simulink subsystem "PID_MotorFB"  (R2024a)
settings: Solver=VariableStepAuto  StartTime=0.0  StopTime=10.0  RelTol=1e-3
undefined symbols (not defined in the file or in its folder): Ki_m, Kp_m, motorFBRate, Tw_m
settings Model: Creator=Peter  LastModifiedBy=Peter

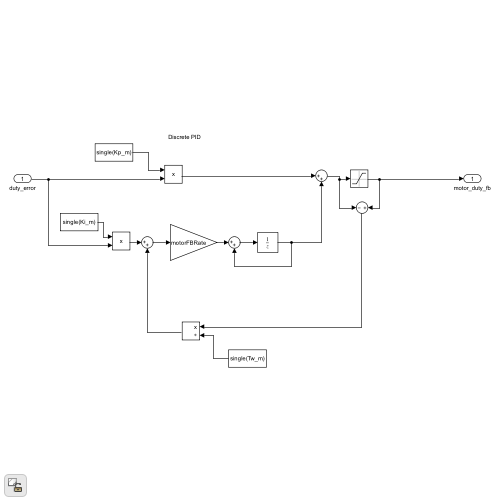
[thumbnail: Simulink's stored preview of the top-level diagram]
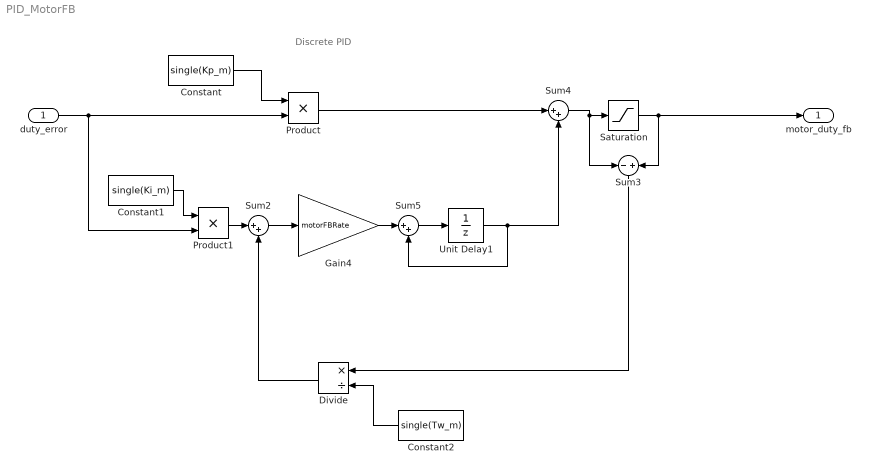
== system PID_MotorFB ==
  note: Discrete PID
  duty_error : Inport
  Constant : Constant  Value=single(Kp_m)
  Constant1 : Constant  Value=single(Ki_m)
  Constant2 : Constant  Value=single(Tw_m)
  Divide : Product  Inputs=*/
  Gain4 : Gain  Gain=motorFBRate
  Product : Product
  Product1 : Product
  Saturation : Saturate  UpperLimit=1  LowerLimit=0
  Sum2 : Sum  Inputs=|++
  Sum3 : Sum  Inputs=-|+
  Sum4 : Sum  Inputs=|++
  Sum5 : Sum  Inputs=|++
  Unit Delay1 : UnitDelay  SampleTime=motorFBRate  HasFrameUpgradeWarning=on
  motor_duty_fb : Outport
  wires:
  Sum5/1 -> Unit Delay1/1
  Unit Delay1/1 -> Sum5/2, Sum4/2
  duty_error/1 -> Product1/2, Product/2
  Saturation/1 -> Sum3/2, motor_duty_fb/1
  Constant/1 -> Product/1
  Sum4/1 -> Saturation/1, Sum3/1
  Gain4/1 -> Sum5/1
  Sum2/1 -> Gain4/1
  Constant1/1 -> Product1/1
  Constant2/1 -> Divide/2
  Product1/1 -> Sum2/1
  Sum3/1 -> Divide/1
  Divide/1 -> Sum2/2
  Product/1 -> Sum4/1
